simulink model "DSBFC_SIM"  (R2024a)
settings: Solver=VariableStepAuto  StartTime=0.0  StopTime=10.0  RelTol=1e-3
libraries: dspfdesign x1
settings Model: Creator=adity  LastModifiedBy=adity

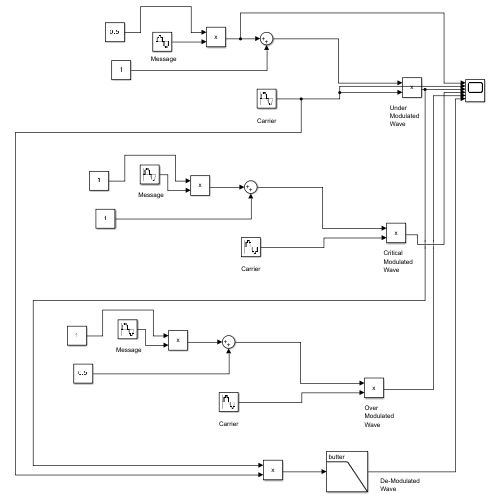
[thumbnail: Simulink's stored preview of the top-level diagram]
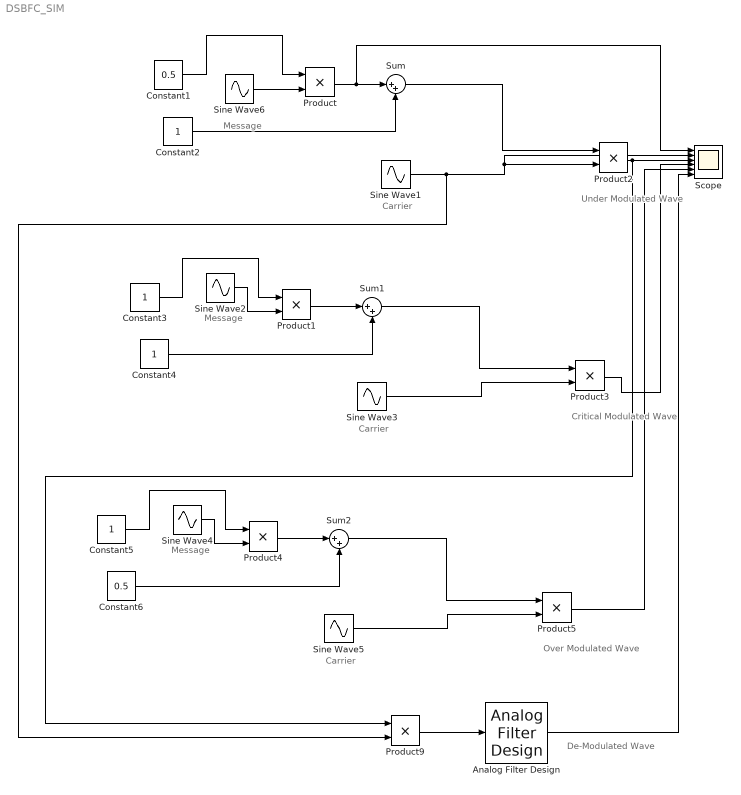
== system DSBFC_SIM ==
  note: Message
  note: Message
  note: Over
      | Modulated
      | Wave
  note: Carrier
  note: Under
      | Modulated
      | Wave
  note: Carrier
  note: Carrier
  note: De-Modulated
      | Wave
  note: Message
  note: Critical
      | Modulated
      | Wave
  Analog Filter Design : dspfdesign/Analog Filter Design  method=Butterworth  filttype=Lowpass  N=8  Wlo=2*pi*10  Whi=80  Rp=2  Rs=40
  Constant1 : Constant  Value=0.5
  Constant{2..5} (4 alike) : Constant
  Constant6 : Constant  Value=0.5
  Product{,1..5,9} (7 alike) : Product
  Scope : Scope  NumInputPorts=6
  Sine Wave1 : Sin  Frequency=2*pi*10  SampleTime=1/1000
  Sine Wave2 : Sin  Frequency=2*pi*1  SampleTime=1/1000
  Sine Wave3 : Sin  Frequency=2*pi*10  SampleTime=1/1000
  Sine Wave4 : Sin  Frequency=2*pi*1  SampleTime=1/1000
  Sine Wave5 : Sin  Frequency=2*pi*10  SampleTime=1/1000
  Sine Wave6 : Sin  Frequency=2*pi*1  SampleTime=1/1000
  Sum : Sum  Inputs=|++
  Sum1 : Sum  Inputs=|++
  Sum2 : Sum  Inputs=|++
  wires:
  Constant2/1 -> Sum/2
  Product/1 -> Scope/1, Sum/1
  Constant1/1 -> Product/1
  Sine Wave2/1 -> Product1/2
  Constant6/1 -> Sum2/2
  Analog Filter Design/1 -> Scope/6
  Sine Wave6/1 -> Product/2
  Product9/1 -> Analog Filter Design/1
  Constant3/1 -> Product1/1
  Product4/1 -> Sum2/1
  Constant5/1 -> Product4/1
  Sum1/1 -> Product3/1
  Product2/1 -> Scope/3, Product9/1
  Sum/1 -> Product2/1
  Sine Wave1/1 -> Scope/2, Product2/2, Product9/2
  Sine Wave5/1 -> Product5/2
  Product5/1 -> Scope/5
  Sum2/1 -> Product5/1
  Constant4/1 -> Sum1/2
  Product3/1 -> Scope/4
  Sine Wave4/1 -> Product4/2
  Sine Wave3/1 -> Product3/2
  Product1/1 -> Sum1/1
